simulink model "withintergral"  (Simulink 7.3)
settings: Solver=ode45  StartTime=0.0  StopTime=50  RelTol=1e-3
model workspace (MAT data in the model file):
  op_withintergral : opcond.OperatingPoint (value not decoded)
libraries: powerlib x1
settings Model: Creator=HP  LastModifiedBy=Twad1
settings OptimizationCC: ExpressionDepthLimit=128
settings DebuggingCC: UnderspecifiedInitializationDetection=Simplified  MergeDetectMultiDrivingBlocksExec=error  SolverPrmCheckMsg=none  StateNameClashWarn=none  StrictBusMsg=ErrorLevel1
settings CodeAppCC: CustomSymbolStrType=$N$R$M_T
settings GRTTargetCC: TargetFunctionLibrary=NOT IN USE  CombineOutputUpdateFcns=on  CPPClassGenCompliant=on

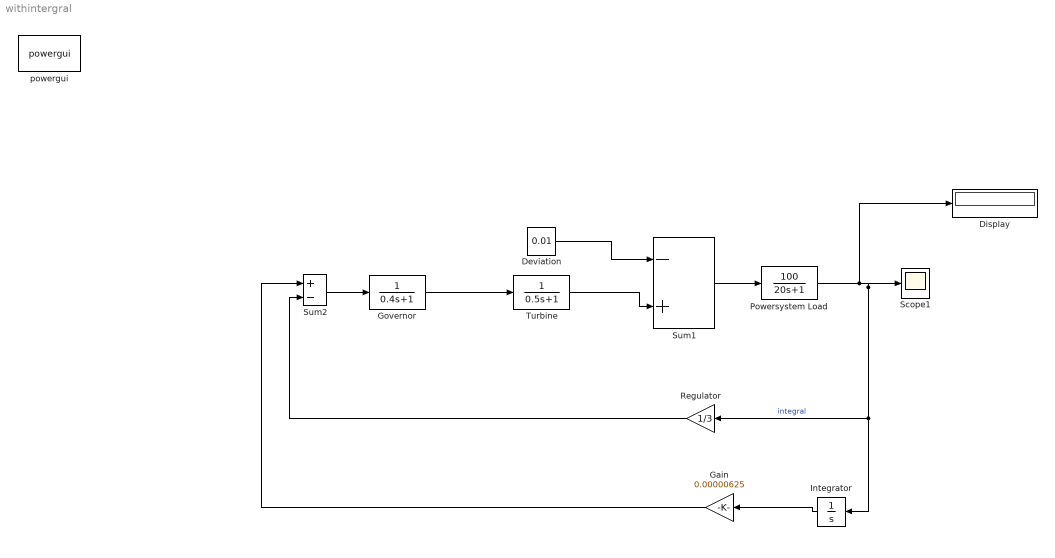
== system withintergral ==
  Deviation : Constant  Value=0.01  OutDataType=fixdt(1, 16)  OutScaling=2^0
  Display : Display
  Gain : Gain  Gain=0.00000625
  Governor : TransferFcn  Denominator=[0.4 1]
  Integrator : Integrator  IgnoreLimit=on
  Powersystem Load : TransferFcn  Numerator=[100]  Denominator=[20 1]
  Regulator : Gain  Gain=1/3
  Scope1 : Scope
      settings: TimeRange=50  YMin=-0.05  YMax=0  SaveName=withintegral  DataFormat=Array
  Sum1 : Sum  Inputs=-+
  Sum2 : Sum  Inputs=+-
  Turbine : TransferFcn  Denominator=[0.5 1]
  powergui : powerlib/powergui  Priority=1  SystemSampleTime=-1  SimulationMode=Continuous  SampleTime=50e-6  frequency=60  SPID=off  DisableSnubberDevices=off  DisableRonSwitches=off  DisableVfSwitches=off  SwTol=0  Interpol=off  frequencyindice=60  echomessages=off  HookPort=off  DisplayEquations=off  FunctionMessages=off  EnableUseOfTLC=off  x0status=blocks  RestoreLinks=warning  Frange=[0:2:500]  Ylog=off  Xlog=on  ShowGrid=off  save=off  variable=ZData  structure=0  ZoomFFT=off  StartTime=0.0  cycles=1  DisplayStyle=1  fundamental=60  FreqAxis=off  MaxFrequency=1000  frequencyindicesteady=1  RmsSteady=1  display=off  Ts=100  methode=off
  wires:
  Governor/1 -> Turbine/1
  Deviation/1 -> Sum1/1
  Turbine/1 -> Sum1/2
  Sum1/1 -> Powersystem Load/1
  Integrator/1 -> Gain/1
  Sum2/1 -> Governor/1
  Gain/1 -> Sum2/1
  Regulator/1 -> Sum2/2
  Powersystem Load/1 -> Integrator/1, Regulator/1, Scope1/1, Display/1  "integral"
